simulink library "SDTlibV1"  (R2025b)
settings: Solver=VariableStepAuto  StartTime=0.0  StopTime=10.0  RelTol=1e-3
PreLoadFcn:
  | addpath(genpath('SDTfct'));
values from neighbouring files (symbols this model uses):
  pass = ra2DCMi(blk.ra)    [view_SDTlib_model.m]
undefined symbols (not defined in the file or in its folder): CMG, DAP0, DPa0, FSM, Ignew, InvDyn, InvDynAug, Jr, KIN, kinematic_model, LS, Mdyn, mnew, mp, OGnew, PMA, ra_norm, RWS, sig4, uls, ureal, uss, uw, XI
libraries: RCTblocks x470, $bdroot x4
(part 3 of 10)

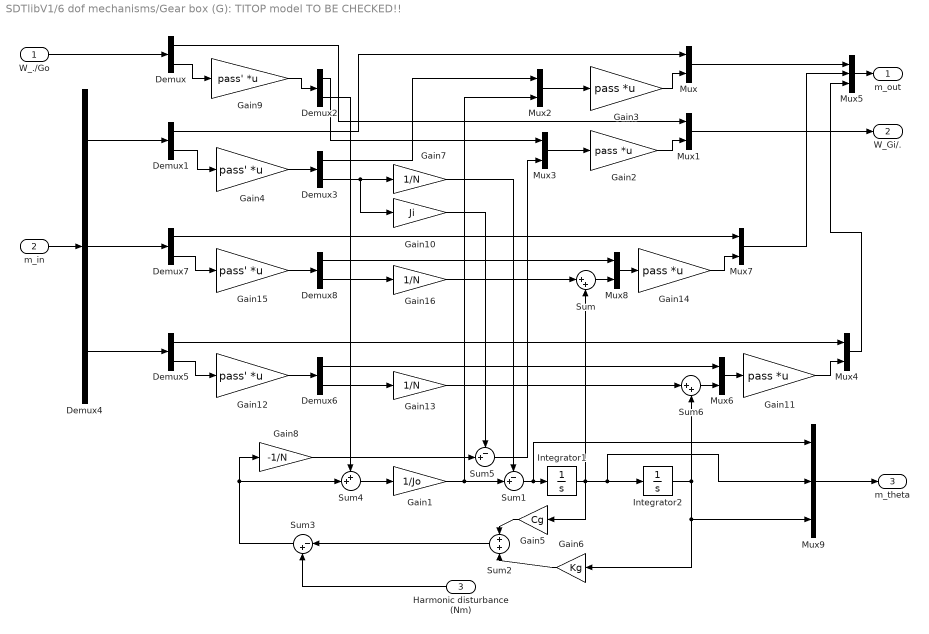
== system SDTlibV1/6 dof mechanisms/Gear box (G): TITOP model TO BE CHECKED!! ==
  W_./Go : Inport  PortDimensions=6
  m_in : Inport  Port=2  PortDimensions=18
  Harmonic disturbance (Nm) : Inport  Port=3
  Demux{,1,5,7} (4 alike) : Demux  Outputs=[3 3]
  Demux{2..3,6,8} (4 alike) : Demux  Outputs=[2 1]
  Demux4 : Demux  Outputs=[6 6 6]
  Gain1 : Gain  Gain=1/Jo
  Gain10 : Gain  Gain=Ji
  Gain{2..3,11,14} (4 alike) : Gain  Gain=pass  Multiplication=Matrix(K*u) (u vector)
  Gain{4,9,12,15} (4 alike) : Gain  Gain=pass'  Multiplication=Matrix(K*u) (u vector)
  Gain13 : Gain  Gain=1/N
  Gain16 : Gain  Gain=1/N
  Gain5 : Gain  Gain=Cg
  Gain6 : Gain  Gain=Kg
  Gain7 : Gain  Gain=1/N
  Gain8 : Gain  Gain=-1/N
  Integrator1 : Integrator
  Integrator2 : Integrator
  Mux{,1,4,7} (4 alike) : Mux  Inputs=[3 3]
  Mux{2..3,6,8} (4 alike) : Mux  Inputs=[2 1]
  Mux5 : Mux  Inputs=[6 6 6]
  Mux9 : Mux  Inputs=3
  Sum : Sum  Inputs=|++
  Sum1 : Sum  Inputs=-+|
  Sum2 : Sum
  Sum3 : Sum  Inputs=|-+
  Sum4 : Sum  Inputs=++|
  Sum5 : Sum  Inputs=-+|
  Sum6 : Sum  Inputs=|++
  m_out : Outport
  W_Gi/. : Outport  Port=2
  m_theta : Outport  Port=3
  wires:
  Mux1/1 -> W_Gi/./1
  Demux1/1 -> Mux/1
  Sum3/1 -> Sum4/2, Gain8/1
  Demux/1 -> Mux1/1
  Gain2/1 -> Mux1/2
  Integrator2/1 -> Mux9/3, Gain6/1, Sum6/2
  Demux/2 -> Gain9/1
  Gain1/1 -> Mux2/2, Sum1/2
  Sum2/1 -> Sum3/1
  Sum4/1 -> Gain1/1
  Gain5/1 -> Sum2/1
  Harmonic disturbance (Nm)/1 -> Sum3/2
  Gain6/1 -> Sum2/2
  Gain3/1 -> Mux/2
  Demux3/2 -> Gain10/1, Gain7/1
  Gain9/1 -> Demux2/1
  Demux2/2 -> Sum4/1
  Mux2/1 -> Gain3/1
  Demux1/2 -> Gain4/1
  Gain4/1 -> Demux3/1
  Mux3/1 -> Gain2/1
  Demux2/1 -> Mux3/1
  Demux3/1 -> Mux2/1
  W_./Go/1 -> Demux/1
  Gain7/1 -> Sum1/1
  Gain8/1 -> Sum5/2
  Sum5/1 -> Mux3/2
  Gain10/1 -> Sum5/1
  Demux4/1 -> Demux1/1
  m_in/1 -> Demux4/1
  Mux/1 -> Mux5/1
  Mux5/1 -> m_out/1
  Integrator1/1 -> Mux9/2, Integrator2/1, Gain5/1, Sum/2
  Demux8/1 -> Mux8/1
  Gain15/1 -> Demux8/1
  Gain14/1 -> Mux7/2
  Demux8/2 -> Gain16/1
  Demux4/2 -> Demux7/1
  Demux7/1 -> Mux7/1
  Demux7/2 -> Gain15/1
  Mux8/1 -> Gain14/1
  Gain16/1 -> Sum/1
  Mux7/1 -> Mux5/2
  Sum/1 -> Mux8/2
  Demux5/2 -> Gain12/1
  Demux6/1 -> Mux6/1
  Mux6/1 -> Gain11/1
  Demux5/1 -> Mux4/1
  Gain11/1 -> Mux4/2
  Gain13/1 -> Sum6/1
  Sum6/1 -> Mux6/2
  Gain12/1 -> Demux6/1
  Demux6/2 -> Gain13/1
  Demux4/3 -> Demux5/1
  Mux4/1 -> Mux5/3
  Mux9/1 -> m_theta/1
  Sum1/1 -> Mux9/1, Integrator1/1

== system SDTlibV1/6 dof mechanisms/Local Spring-Damper system  ==
  m_C : Inport  PortDimensions=18
  m_P : Inport  Port=2  PortDimensions=18
  Damping Matrix : RCTblocks/Uncertain State Space  Tag=USS  USystem=ss(D_O)  UValue=[]  X0=[]  uX0=[]
  Damping Matrix1 : RCTblocks/Uncertain State Space  Tag=USS  USystem=ss(K_O)  UValue=[]  X0=[]  uX0=[]
  Demux : Demux  Outputs=[6 6 6]
  Demux1 : Demux  Outputs=[6 6 6]
  Kinematic model between O and C : RCTblocks/Uncertain State Space  Tag=USS  USystem=ss(TAU_OC)  UValue=[]  X0=[]  uX0=[]
  Kinematic model between O and C' : RCTblocks/Uncertain State Space  Tag=USS  USystem=ss(TAU_OC')  UValue=[]  X0=[]  uX0=[]
  Kinematic model between O and C1 : RCTblocks/Uncertain State Space  Tag=USS  USystem=ss(TAU_OC)  UValue=[]  X0=[]  uX0=[]
  Kinematic model between O and P : RCTblocks/Uncertain State Space  Tag=USS  USystem=ss(TAU_OP)  UValue=[]  X0=[]  uX0=[]
  Kinematic model between O and P' : RCTblocks/Uncertain State Space  Tag=USS  USystem=ss(TAU_OP')  UValue=[]  X0=[]  uX0=[]
  Kinematic model between O and P1 : RCTblocks/Uncertain State Space  Tag=USS  USystem=ss(TAU_OP)  UValue=[]  X0=[]  uX0=[]
  Sum : Sum  Inputs=|+-
  Sum1 : Sum  Inputs=++|
  Sum2 : Sum  Inputs=|+-
  Terminator : Terminator
  Terminator1 : Terminator
  W(./s,C) : Outport  VectorParamsAs1DForOutWhenUnconnected=off
  W(s/.,P) : Outport  Port=2  VectorParamsAs1DForOutWhenUnconnected=off
  wires:
  Kinematic model between O and C'/1 -> W(./s,C)/1
  Kinematic model between O and P'/1 -> W(s/.,P)/1
  Sum/1 -> Damping Matrix/1
  Kinematic model between O and C/1 -> Sum/1
  Kinematic model between O and P/1 -> Sum/2
  Damping Matrix/1 -> Sum1/2
  Damping Matrix1/1 -> Sum1/1
  Sum2/1 -> Damping Matrix1/1
  Sum1/1 -> Kinematic model between O and C'/1, Kinematic model between O and P'/1
  m_P/1 -> Demux/1
  Demux/2 -> Kinematic model between O and P/1
  Demux/1 -> Terminator/1
  m_C/1 -> Demux1/1
  Demux1/1 -> Terminator1/1
  Demux1/2 -> Kinematic model between O and C/1
  Demux1/3 -> Kinematic model between O and C1/1
  Demux/3 -> Kinematic model between O and P1/1
  Kinematic model between O and C1/1 -> Sum2/1
  Kinematic model between O and P1/1 -> Sum2/2

== system SDTlibV1/6 dof mechanisms/PMA ==
  m_P : Inport
  u_PMA : Inport  Port=2
  Demux : Demux  Outputs=[6 12]
  Multi port rigid body : Subsystem  mask(Multi-port rigid body (6nx6n)){m=Mc-mp, Ig=IatG, OG=PG, n=2, numinv=1, OP1=[0;0;0], OP2=PG, OP3=[ureal('P3_y',1,'percent',10);0;0], OP4=[0;0;0], OP5=[0;0;0]}
      mask prompts: m "Mass (Kg)"; Ig "Inertia (at G, Kg m^2)"; OG "OG (3x1 vector, m)"; n "Number of ports"; numinv "Port to be inverted"; OP1 "OP1 (3x1 vector, m)"; OP2 "OP2 (3x1 vector, m)"; OP3 "OP3 (3x1 vector, m)"; OP4 "OP4 (3x1 vector, m)"; OP5 "OP5 (3x1 vector,m)"
      mask help:
      | 6nx6n dynamic model of a rigid body at n given points (ports) between wrenches applied at the n points (input) and acceleration twists at these points (output).
      |
      | 0: the reference point
      | G: the center of mass
      | Pi (i=1:n): the n given connection points (n<6).
      |
      | All parameters are expressed in the body frame.
      | Each parameter can be an uncertain parameter declared with "ureal"
      |
      | The 6x6 channel associated to one port can be inverted: then the input of this channel is the acceleration twist imposed at this point and the output is the wrench applied by this body.
      mask init:
      | MultiPortRigidBodyAug
      mask Help: web('Docmultiportrigidbody.html','-browser','-browser')
      mask TypeOptions n: 1 | 2 | 3 | 4 | 5
      mask TypeOptions numinv: 1 | 2 | 3 | 4 | 5
      mask DialogControl ParameterGroupVar Prompt: Main parameters
      mask DialogControl port1 Prompt: Port #1
      mask DialogControl port2 Prompt: #2
      mask DialogControl port3 Prompt: #3
      mask DialogControl port4 Prompt: #4
      mask DialogControl port5 Prompt: #5
      mask Display:
      | disp('Multi-port\n rigid body\n [18(n-1)+6]x[6(n-1)+18])')
      | if n==1,
      |     if numinv==1,
      |         port_label('input', 1,'m_P')
      |         port_label('output',1,'W_body/.,P')
      |     else
      |         port_label('input', 1,'W_./body,P')
      |         port_label('output',1,'m_P')
      |     end
      | else
      |     for ii=1:n
      |         if numinv==ii,
      |             port_label('output',ii,['W_body/.,P',num2str(ii)])
      |             port_label('input', ii,['m_P',num2str(ii)])
      |         else
      |             port_label('input', ii,['W_./body,P',num2str(ii)])
      |             port_label('output',ii,['m_P',num2str(ii)])
      |         end
      |     end
      | end
  Terminator : Terminator
  proof mass : Subsystem  mask(Mass-spring-model model(6x6)){v=v, m=mp, k=k, d=d}
      mask prompts: v "v (3x1 vector)"; m "mass (Kg)"; k "stiffness (N/m)"; d "damper (Ns/m)"
      mask help:
      | Simplified dynamic model of a spring-mass-damper model located at point P (connection point with the hub):
      | 6x6 transfer between acceleretion twist at P and wrench applied by the spring-mass system at P. The model is expressed in the (inherit) body frame.
      |
      | v: the direction vector of the spring-mass system.
      | Each parameter (except v) can be an uncertain parameter declared with "ureal"
      mask init:
      | pass=ra2DCMi(v);
      mask DialogControl ParameterGroupVar Prompt: Main parameters
      mask Display:
      | disp('1D \n mass-spring-damper \n model(6x6)')
      | port_label('input', 1, 'Xddot')
      | port_label('output', 1, 'W_body/.')
      | port_label('input', 2, 'u_PMA')
      | port_label('output', 2, 'x_PMA')
  W_body/.,P : Outport
  x_PMA : Outport  Port=2
  wires:
  Multi port rigid body/1(out1) -> W_body/.,P/1
  u_PMA/1 -> proof mass/2(u_PMA)
  m_P/1 -> Multi port rigid body/1(in1)
  proof mass/1(W_body/.) -> Multi port rigid body/2(in2)
  proof mass/2(x_PMA) -> x_PMA/1
  Multi port rigid body/2(out2) -> Demux/1
  Demux/1 -> proof mass/1(Xddot)
  Demux/2 -> Terminator/1

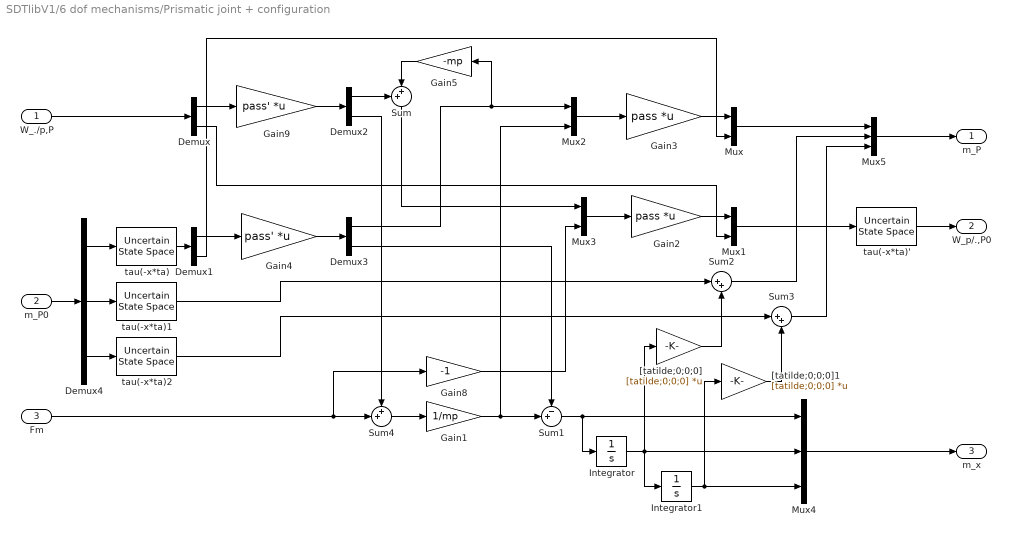
== system SDTlibV1/6 dof mechanisms/Prismatic joint + configuration ==
  W_./p,P : Inport  PortDimensions=6
  m_P0 : Inport  Port=2  PortDimensions=18
  Fm : Inport  Port=3  PortDimensions=1
  Demux : Demux  Outputs=[3 3]
  Demux1 : Demux  Outputs=[3 3]
  Demux2 : Demux  Outputs=[2 1]
  Demux3 : Demux  Outputs=[2 1]
  Demux4 : Demux  Outputs=[6 6 6]
  Gain1 : Gain  Gain=1/mp
  Gain2 : Gain  Gain=pass  Multiplication=Matrix(K*u) (u vector)
  Gain3 : Gain  Gain=pass  Multiplication=Matrix(K*u) (u vector)
  Gain4 : Gain  Gain=pass'  Multiplication=Matrix(K*u) (u vector)
  Gain5 : Gain  Gain=-mp
  Gain8 : Gain  Gain=-1
  Gain9 : Gain  Gain=pass'  Multiplication=Matrix(K*u) (u vector)
  Integrator : Integrator
  Integrator1 : Integrator
  Mux : Mux  Inputs=[3 3]
  Mux1 : Mux  Inputs=[3 3]
  Mux2 : Mux  Inputs=[2 1]
  Mux3 : Mux  Inputs=[2 1]
  Mux4 : Mux  Inputs=3
  Mux5 : Mux  Inputs=[6 6 6]
  Sum : Sum  Inputs=++|
  Sum1 : Sum  Inputs=-+|
  Sum2 : Sum  Inputs=|++
  Sum3 : Sum  Inputs=|++
  Sum4 : Sum  Inputs=++|
  "[tatilde;0;0;0]" : Gain  Gain=[tatilde;0;0;0]  Multiplication=Matrix(K*u) (u vector)
  "[tatilde;0;0;0]1" : Gain  Gain=[tatilde;0;0;0]  Multiplication=Matrix(K*u) (u vector)
  tau(-x*ta) : RCTblocks/Uncertain State Space  Tag=USS  USystem=tau_x  UValue=[]  X0=[]  uX0=[]
  tau(-x*ta)' : RCTblocks/Uncertain State Space  Tag=USS  USystem=tau_x'  UValue=[]  X0=[]  uX0=[]
  tau(-x*ta)1 : RCTblocks/Uncertain State Space  Tag=USS  USystem=tau_x  UValue=[]  X0=[]  uX0=[]
  tau(-x*ta)2 : RCTblocks/Uncertain State Space  Tag=USS  USystem=tau_x  UValue=[]  X0=[]  uX0=[]
  m_P : Outport  VectorParamsAs1DForOutWhenUnconnected=off
  W_p/.,P0 : Outport  Port=2  VectorParamsAs1DForOutWhenUnconnected=off
  m_x : Outport  Port=3  VectorParamsAs1DForOutWhenUnconnected=off
  wires:
  Mux1/1 -> tau(-x*ta)'/1
  Fm/1 -> Gain8/1, Sum4/2
  Gain1/1 -> Mux2/2, Sum1/2
  Sum4/1 -> Gain1/1
  Demux3/2 -> Sum1/1
  Gain9/1 -> Demux2/1
  Mux2/1 -> Gain3/1
  Gain4/1 -> Demux3/1
  Mux3/1 -> Gain2/1
  Gain8/1 -> Mux3/2
  Demux3/1 -> Gain5/1, Mux2/1
  W_./p,P/1 -> Demux/1
  Demux/1 -> Gain9/1
  Demux2/2 -> Sum4/1
  Gain2/1 -> Mux1/1
  Demux/2 -> Mux1/2
  Demux1/1 -> Gain4/1
  Demux1/2 -> Mux/2
  Gain3/1 -> Mux/1
  tau(-x*ta)/1 -> Demux1/1
  tau(-x*ta)'/1 -> W_p/.,P0/1
  Demux2/1 -> Sum/1
  Gain5/1 -> Sum/2
  Sum/1 -> Mux3/1
  Demux4/1 -> tau(-x*ta)/1
  Demux4/2 -> tau(-x*ta)1/1
  Demux4/3 -> tau(-x*ta)2/1
  m_P0/1 -> Demux4/1
  Mux4/1 -> m_x/1
  "[tatilde;0;0;0]1"/1 -> Sum3/2
  "[tatilde;0;0;0]"/1 -> Sum2/2
  Integrator1/1 -> "[tatilde;0;0;0]1"/1, Mux4/3
  Integrator/1 -> "[tatilde;0;0;0]"/1, Mux4/2, Integrator1/1
  Sum1/1 -> Integrator/1, Mux4/1
  tau(-x*ta)1/1 -> Sum2/1
  tau(-x*ta)2/1 -> Sum3/1
  Mux/1 -> Mux5/1
  Sum2/1 -> Mux5/2
  Sum3/1 -> Mux5/3
  Mux5/1 -> m_P/1

== system SDTlibV1/6 dof mechanisms/RW ==
  m : Inport  PortDimensions=18
  u (Nm) : Inport  Port=2  PortDimensions=1
  Demux : Demux  Outputs=[3 3]
  Demux1 : Demux  Outputs=[2 1]
  Demux2 : Demux  Outputs=[6 6 6]
  Demux3 : Demux  Outputs=[3 3]
  Demux4 : Demux  Outputs=[2 1]
  Gain : Gain  Gain=-1
  Gain1 : Gain  Gain=pass'  Multiplication=Matrix(K*u) (u vector)
  Gain10 : Gain  Gain=pass'  Multiplication=Matrix(K*u) (u vector)
  Gain2 : Gain  Gain=pass  Multiplication=Matrix(K*u) (u vector)
  Gain3 : Gain  Gain=m*eye(3)  Multiplication=Matrix(K*u) (u vector)
  Gain4 : Gain  Gain=diag([Ir Ir 0])  Multiplication=Matrix(K*u) (u vector)
  Gain5 : Gain  Gain=Tau_GP  Multiplication=Matrix(K*u) (u vector)
  Gain6 : Gain  Gain=[0 Iw;-Iw 0]  Multiplication=Matrix(K*u) (u vector)
  Gain7 : Gain  Gain=1/Iw
  Gain8 : Gain  Gain=-Tau_GP'  Multiplication=Matrix(K*u) (u vector)
  Gain9 : Gain  Gain=Tau_GP  Multiplication=Matrix(K*u) (u vector)
  Mux : Mux  Inputs=[3 3]
  Mux2 : Mux  Inputs=[2 1]
  Omega : RCTblocks/Uncertain State Space  Tag=USS  USystem=uss(Omega*eye(2))  UValue=[]  X0=[]  uX0=[]
  Sum : Sum
  Sum1 : Sum  Inputs=-+|
  Terminator{,1..3} (4 alike) : Terminator
  W_body/. : Outport  VectorParamsAs1DForOutWhenUnconnected=off
  Omega dot (rad/s^2) : Outport  Port=2  PortDimensions=1  VectorParamsAs1DForOutWhenUnconnected=off
  wires:
  Gain3/1 -> Mux/1
  Gain2/1 -> Mux/2
  Demux/1 -> Gain3/1
  Demux/2 -> Gain1/1
  Gain4/1 -> Sum/1
  Sum/1 -> Gain2/1
  Gain1/1 -> Demux1/1, Gain4/1
  Demux4/1 -> Gain6/1
  Gain6/1 -> Omega/1
  Gain8/1 -> W_body/./1
  Mux/1 -> Gain8/1
  Gain9/1 -> Demux/1
  u (Nm)/1 -> Gain/1
  Sum1/1 -> Omega dot (rad/s^2)/1
  Gain7/1 -> Sum1/2
  Gain/1 -> Mux2/2, Gain7/1
  Omega/1 -> Mux2/1
  Mux2/1 -> Sum/2
  Demux2/1 -> Gain9/1
  m/1 -> Demux2/1
  Demux2/2 -> Gain5/1
  Gain5/1 -> Demux3/1
  Demux3/2 -> Gain10/1
  Demux3/1 -> Terminator/1
  Demux2/3 -> Terminator1/1
  Demux1/2 -> Sum1/1
  Demux1/1 -> Terminator2/1
  Gain10/1 -> Demux4/1
  Demux4/2 -> Terminator3/1

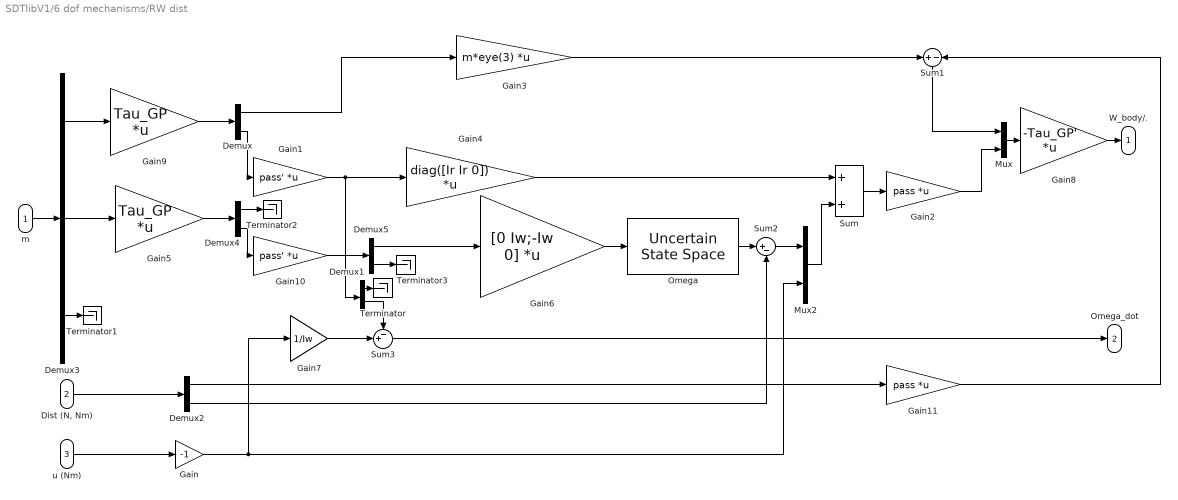
== system SDTlibV1/6 dof mechanisms/RW dist ==
  m : Inport  PortDimensions=18
  "Dist (N, Nm)    " : Inport  Port=2
  u (Nm) : Inport  Port=3  PortDimensions=1
  Demux : Demux  Outputs=[3 3]
  Demux1 : Demux  Outputs=[2 1]
  Demux2 : Demux  Outputs=[3 2]
  Demux3 : Demux  Outputs=[6 6 6]
  Demux4 : Demux  Outputs=[3 3]
  Demux5 : Demux  Outputs=[2 1]
  Gain : Gain  Gain=-1
  Gain1 : Gain  Gain=pass'  Multiplication=Matrix(K*u) (u vector)
  Gain10 : Gain  Gain=pass'  Multiplication=Matrix(K*u) (u vector)
  Gain11 : Gain  Gain=pass  Multiplication=Matrix(K*u) (u vector)
  Gain2 : Gain  Gain=pass  Multiplication=Matrix(K*u) (u vector)
  Gain3 : Gain  Gain=m*eye(3)  Multiplication=Matrix(K*u) (u vector)
  Gain4 : Gain  Gain=diag([Ir Ir 0])  Multiplication=Matrix(K*u) (u vector)
  Gain5 : Gain  Gain=Tau_GP  Multiplication=Matrix(K*u) (u vector)
  Gain6 : Gain  Gain=[0 Iw;-Iw 0]  Multiplication=Matrix(K*u) (u vector)
  Gain7 : Gain  Gain=1/Iw
  Gain8 : Gain  Gain=-Tau_GP'  Multiplication=Matrix(K*u) (u vector)
  Gain9 : Gain  Gain=Tau_GP  Multiplication=Matrix(K*u) (u vector)
  Mux : Mux  Inputs=[3 3]
  Mux2 : Mux  Inputs=[2 1]
  Omega : RCTblocks/Uncertain State Space  Tag=USS  USystem=uss(Omega*eye(2))  UValue=[]  X0=[]  uX0=[]
  Sum : Sum
  Sum1 : Sum  Inputs=+-
  Sum2 : Sum  Inputs=|+-
  Sum3 : Sum  Inputs=-+|
  Terminator{,1..3} (4 alike) : Terminator
  W_body/. : Outport  VectorParamsAs1DForOutWhenUnconnected=off
  Omega_dot : Outport  Port=2  PortDimensions=1  VectorParamsAs1DForOutWhenUnconnected=off
  wires:
  Sum3/1 -> Omega_dot/1
  Gain7/1 -> Sum3/2
  Mux2/1 -> Sum/2
  Sum2/1 -> Mux2/1
  Omega/1 -> Sum2/1
  Gain/1 -> Gain7/1, Mux2/2
  u (Nm)/1 -> Gain/1
  Sum1/1 -> Mux/1
  Gain11/1 -> Sum1/2
  Gain3/1 -> Sum1/1
  Demux2/2 -> Sum2/2
  "Dist (N, Nm)    "/1 -> Demux2/1
  Demux2/1 -> Gain11/1
  Gain9/1 -> Demux/1
  Mux/1 -> Gain8/1
  Gain8/1 -> W_body/./1
  Gain6/1 -> Omega/1
  Demux5/1 -> Gain6/1
  Gain1/1 -> Gain4/1, Demux1/1
  Sum/1 -> Gain2/1
  Gain4/1 -> Sum/1
  Demux/2 -> Gain1/1
  Demux/1 -> Gain3/1
  Gain2/1 -> Mux/2
  Demux3/1 -> Gain9/1
  m/1 -> Demux3/1
  Demux3/2 -> Gain5/1
  Demux1/2 -> Sum3/1
  Demux1/1 -> Terminator/1
  Demux3/3 -> Terminator1/1
  Demux4/2 -> Gain10/1
  Gain5/1 -> Demux4/1
  Demux4/1 -> Terminator2/1
  Gain10/1 -> Demux5/1
  Demux5/2 -> Terminator3/1

== system SDTlibV1/6 dof mechanisms/RW_NL ==
  m : Inport  PortDimensions=18
  u (Nm) : Inport  Port=2  PortDimensions=1
  Demux : Demux  Outputs=[3 3]
  Demux1 : Demux  Outputs=[2 1]
  Demux2 : Demux  Outputs=[6 6 6]
  Demux3 : Demux  Outputs=[3 3]
  Demux4 : Demux  Outputs=[2 1]
  Gain : Gain  Gain=-1
  Gain1 : Gain  Gain=pass'  Multiplication=Matrix(K*u) (u vector)
  Gain10 : Gain  Gain=Tau_GP  Multiplication=Matrix(K*u) (u vector)
  Gain2 : Gain  Gain=pass  Multiplication=Matrix(K*u) (u vector)
  Gain3 : Gain  Gain=m*eye(3)  Multiplication=Matrix(K*u) (u vector)
  Gain4 : Gain  Gain=diag([Ir Ir 0])  Multiplication=Matrix(K*u) (u vector)
  Gain5 : Gain  Gain=pass'  Multiplication=Matrix(K*u) (u vector)
  Gain6 : Gain  Gain=[0 Iw;-Iw 0]  Multiplication=Matrix(K*u) (u vector)
  Gain7 : Gain  Gain=1/Iw
  Gain8 : Gain  Gain=-Tau_GP'  Multiplication=Matrix(K*u) (u vector)
  Gain9 : Gain  Gain=Tau_GP  Multiplication=Matrix(K*u) (u vector)
  Integrator2 : Integrator  InitialCondition=Omega
  Mux : Mux  Inputs=[3 3]
  Mux2 : Mux  Inputs=[2 1]
  Product : Product
  Sum : Sum
  Sum1 : Sum  Inputs=-+
  Terminator{,1..3} (4 alike) : Terminator
  W_body/. : Outport  VectorParamsAs1DForOutWhenUnconnected=off
  Omega : Outport  Port=2  PortDimensions=1  VectorParamsAs1DForOutWhenUnconnected=off
  wires:
  Mux2/1 -> Sum/2
  Product/1 -> Mux2/1
  Demux1/2 -> Sum1/1
  Gain7/1 -> Sum1/2
  Sum1/1 -> Integrator2/1
  Gain/1 -> Gain7/1, Mux2/2
  Integrator2/1 -> Product/2, Omega/1
  u (Nm)/1 -> Gain/1
  Gain9/1 -> Demux/1
  Mux/1 -> Gain8/1
  Gain8/1 -> W_body/./1
  Gain6/1 -> Product/1
  Demux4/1 -> Gain6/1
  Gain1/1 -> Gain4/1, Demux1/1
  Sum/1 -> Gain2/1
  Gain4/1 -> Sum/1
  Demux/2 -> Gain1/1
  Demux/1 -> Gain3/1
  Gain2/1 -> Mux/2
  Gain3/1 -> Mux/1
  Demux2/1 -> Gain9/1
  m/1 -> Demux2/1
  Demux1/1 -> Terminator/1
  Demux2/3 -> Terminator1/1
  Gain5/1 -> Demux4/1
  Gain10/1 -> Demux3/1
  Demux3/2 -> Gain5/1
  Demux2/2 -> Gain10/1
  Demux3/1 -> Terminator2/1
  Demux4/2 -> Terminator3/1

== system SDTlibV1/6 dof mechanisms/Revolute joint ==
  W_./r_out : Inport  PortDimensions=6
  m_in : Inport  Port=2  PortDimensions=18
  Cm : Inport  Port=3  PortDimensions=1
  Demux : Demux  Outputs=[3 3]
  Demux1 : Demux  Outputs=[3 3]
  Demux2 : Demux  Outputs=[2 1]
  Demux3 : Demux  Outputs=[2 1]
  Demux4 : Demux  Outputs=[6 6 6]
  Gain1 : Gain  Gain=1/Jr
  Gain2 : Gain  Gain=pass  Multiplication=Matrix(K*u) (u vector)
  Gain3 : Gain  Gain=pass  Multiplication=Matrix(K*u) (u vector)
  Gain4 : Gain  Gain=pass'  Multiplication=Matrix(K*u) (u vector)
  Gain8 : Gain  Gain=-1
  Gain9 : Gain  Gain=pass'  Multiplication=Matrix(K*u) (u vector)
  Integrator : Integrator
  Integrator1 : Integrator
  Mux : Mux  Inputs=[3 3]
  Mux1 : Mux  Inputs=[3 3]
  Mux2 : Mux  Inputs=[2 1]
  Mux3 : Mux  Inputs=[2 1]
  Mux4 : Mux  Inputs=3
  Mux5 : Mux  Inputs=[6 6 6]
  Sum : Sum  Inputs=|++
  Sum1 : Sum  Inputs=-+|
  Sum2 : Sum  Inputs=|++
  Sum4 : Sum  Inputs=++|
  "[0;0;0;ran]" : Gain  Gain=[zeros(3,1);ran]  Multiplication=Matrix(K*u) (u vector)
  "[0;0;0;ran]1" : Gain  Gain=[zeros(3,1);ran]  Multiplication=Matrix(K*u) (u vector)
  m_out : Outport  VectorParamsAs1DForOutWhenUnconnected=off
  W_r_in/. : Outport  Port=2  VectorParamsAs1DForOutWhenUnconnected=off
  m_theta : Outport  Port=3  VectorParamsAs1DForOutWhenUnconnected=off
  wires:
  Mux1/1 -> W_r_in/./1
  Demux1/1 -> Mux/1
  Cm/1 -> Gain8/1, Sum4/2
  Demux/1 -> Mux1/1
  Gain2/1 -> Mux1/2
  Sum1/1 -> Integrator/1, Mux4/1
  Demux/2 -> Gain9/1
  Gain1/1 -> Mux2/2, Sum1/2
  Sum4/1 -> Gain1/1
  Gain3/1 -> Mux/2
  Demux3/2 -> Sum1/1
  Gain9/1 -> Demux2/1
  Demux2/2 -> Sum4/1
  Mux2/1 -> Gain3/1
  Demux1/2 -> Gain4/1
  Gain4/1 -> Demux3/1
  Mux3/1 -> Gain2/1
  Gain8/1 -> Mux3/2
  Demux2/1 -> Mux3/1
  Demux3/1 -> Mux2/1
  W_./r_out/1 -> Demux/1
  Demux4/1 -> Demux1/1
  m_in/1 -> Demux4/1
  Integrator/1 -> "[0;0;0;ran]"/1, Mux4/2, Integrator1/1
  Integrator1/1 -> "[0;0;0;ran]1"/1, Mux4/3
  Mux4/1 -> m_theta/1
  Demux4/2 -> Sum/1
  "[0;0;0;ran]"/1 -> Sum/2
  "[0;0;0;ran]1"/1 -> Sum2/2
  Demux4/3 -> Sum2/1
  Mux/1 -> Mux5/1
  Sum/1 -> Mux5/2
  Sum2/1 -> Mux5/3
  Mux5/1 -> m_out/1

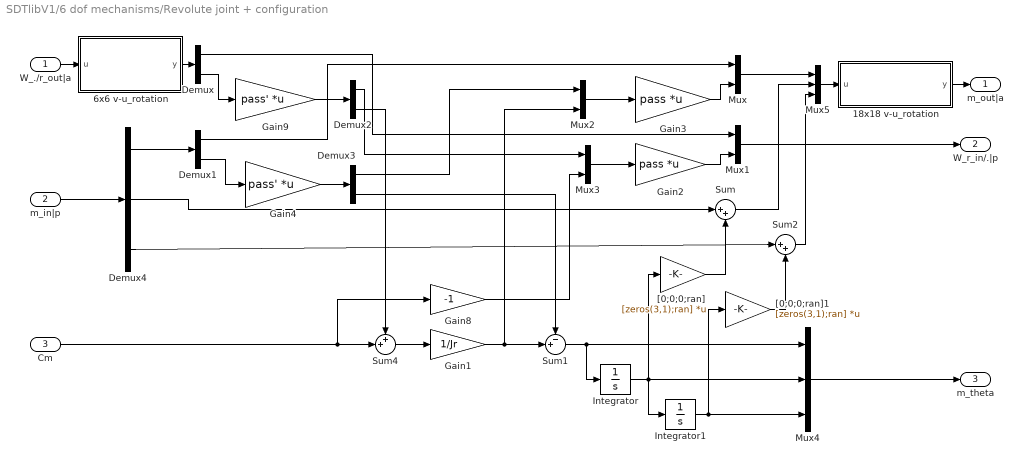
== system SDTlibV1/6 dof mechanisms/Revolute joint + configuration ==
  W_./r_out|a : Inport  PortDimensions=6
  m_in|p : Inport  Port=2  PortDimensions=18
  Cm : Inport  Port=3  PortDimensions=1
  18x18 v-u_rotation : Subsystem  mask(18x18 rotation matrix (around a given axis)){ra=ra, theta=theta, transp=on}
      mask prompts: ra "Rotation axis (3x1 vector)"; theta "Angle (rad)"; transp "Matrix transposed"
      mask help:
      | For 6 d.o.f. body motion vector (3 translations and 3 rotations, acceleration velocities and positions), this block Implement the 18x18 rotation matrix (or its transposed)  for a given angle around a given axis.
      |
      | Angle  (rad) can be an uncertain parameter declared with "ureal" with mode 'Range'
      | Ex: ureal('NAME',0,'Range',[-pi pi])
      | Then, ULINEARIZE will provide a model involving the block named "tan_NAME_div4".
      mask init:
      | vUrotation3x3
      mask Help: web('Doc6vurotation.html','-browser','-browser')
      mask Display:
      | disp('v-rot\n18x18')
      | if transp
      |     port_label('input', 1, '[.]_R1')
      |     port_label('output', 1, '[.]_R2')
      | else
      |     port_label('input', 1, '[.]_R2')
      |     port_label('output', 1, '[.]_R1')
      | end
  6x6 v-u_rotation : Subsystem  mask(6x6 rotation matrix (around a given axis)){ra=ra, theta=theta, transp=off}
      mask prompts: ra "Rotation axis (3x1 vector)"; theta "Angle (rad)"; transp "Matrix transposed"
      mask help:
      | For 6 d.o.f. body motion (3 translations and 3 rotations), this block Implement the 6x6 rotation matrix (or its transposed) for a given angle around a given axis.
      |
      | Angle  (rad) can be an uncertain parameter declared with "ureal" with mode 'Range'
      | Ex: ureal('NAME',0,'Range',[-pi pi])
      | Then, ULINEARIZE will provide a model involving the block named "tan_NAME_div4".
      mask init:
      | vUrotation3x3
      mask Help: web('Doc6vurotation.html','-browser','-browser')
      mask Display:
      | disp('v-rot\n6x6')
      | if transp
      |     port_label('input', 1, '[.]_R1')
      |     port_label('output', 1, '[.]_R2')
      | else
      |     port_label('input', 1, '[.]_R2')
      |     port_label('output', 1, '[.]_R1')
      | end
  Demux : Demux  Outputs=[3 3]
  Demux1 : Demux  Outputs=[3 3]
  Demux2 : Demux  Outputs=[2 1]
  Demux3 : Demux  Outputs=[2 1]
  Demux4 : Demux  Outputs=[6 6 6]
  Gain1 : Gain  Gain=1/Jr
  Gain2 : Gain  Gain=pass  Multiplication=Matrix(K*u) (u vector)
  Gain3 : Gain  Gain=pass  Multiplication=Matrix(K*u) (u vector)
  Gain4 : Gain  Gain=pass'  Multiplication=Matrix(K*u) (u vector)
  Gain8 : Gain  Gain=-1
  Gain9 : Gain  Gain=pass'  Multiplication=Matrix(K*u) (u vector)
  Integrator : Integrator
  Integrator1 : Integrator
  Mux : Mux  Inputs=[3 3]
  Mux1 : Mux  Inputs=[3 3]
  Mux2 : Mux  Inputs=[2 1]
  Mux3 : Mux  Inputs=[2 1]
  Mux4 : Mux  Inputs=3
  Mux5 : Mux  Inputs=[6 6 6]
  Sum : Sum  Inputs=|++
  Sum1 : Sum  Inputs=-+|
  Sum2 : Sum  Inputs=|++
  Sum4 : Sum  Inputs=++|
  "[0;0;0;ran]" : Gain  Gain=[zeros(3,1);ran]  Multiplication=Matrix(K*u) (u vector)
  "[0;0;0;ran]1" : Gain  Gain=[zeros(3,1);ran]  Multiplication=Matrix(K*u) (u vector)
  m_out|a : Outport  VectorParamsAs1DForOutWhenUnconnected=off
  W_r_in/.|p : Outport  Port=2  VectorParamsAs1DForOutWhenUnconnected=off
  m_theta : Outport  Port=3  VectorParamsAs1DForOutWhenUnconnected=off
  wires:
  18x18 v-u_rotation/1(y) -> m_out|a/1
  6x6 v-u_rotation/1(y) -> Demux/1
  Demux3/1 -> Mux2/1
  Demux2/1 -> Mux3/1
  Gain8/1 -> Mux3/2
  Mux3/1 -> Gain2/1
  Gain4/1 -> Demux3/1
  Demux1/2 -> Gain4/1
  Mux2/1 -> Gain3/1
  Demux2/2 -> Sum4/1
  Gain9/1 -> Demux2/1
  Demux3/2 -> Sum1/1
  Gain3/1 -> Mux/2
  Sum4/1 -> Gain1/1
  Gain1/1 -> Sum1/2, Mux2/2
  Demux/2 -> Gain9/1
  Gain2/1 -> Mux1/2
  Demux/1 -> Mux1/1
  Cm/1 -> Sum4/2, Gain8/1
  Demux1/1 -> Mux/1
  Mux1/1 -> W_r_in/.|p/1
  W_./r_out|a/1 -> 6x6 v-u_rotation/1(u)
  Demux4/1 -> Demux1/1
  m_in|p/1 -> Demux4/1
  Integrator/1 -> "[0;0;0;ran]"/1, Mux4/2, Integrator1/1
  Mux4/1 -> m_theta/1
  Sum1/1 -> Integrator/1, Mux4/1
  Integrator1/1 -> "[0;0;0;ran]1"/1, Mux4/3
  "[0;0;0;ran]"/1 -> Sum/2
  "[0;0;0;ran]1"/1 -> Sum2/2
  Demux4/2 -> Sum/1
  Demux4/3 -> Sum2/1
  Mux/1 -> Mux5/1
  Mux5/1 -> 18x18 v-u_rotation/1(u)
  Sum/1 -> Mux5/2
  Sum2/1 -> Mux5/3

== system SDTlibV1/6 dof mechanisms/u_sloshing ==
  m : Inport  PortDimensions=18
  -m1 : RCTblocks/Uncertain State Space  Tag=USS  USystem=uss(-m*eye(3))  UValue=[]  X0=[]  uX0=[]
  2*xi : RCTblocks/Uncertain State Space  Tag=USS  USystem=uss(2*xi)  UValue=[]  X0=[]  uX0=[]
  Add1 : Sum
  Add3 : Sum  Inputs=+-
  Demux : Demux  Outputs=[3 3]
  Demux1 : Demux  Outputs=[2 1]
  Demux2 : Demux  Outputs=[6 12]
  Gain2 : Gain  Gain=pass'  Multiplication=Matrix(K*u) (u vector)
  Gain3 : Gain  Gain=pass  Multiplication=Matrix(K*u) (u vector)
  Ground : Ground
  Integrator : Integrator
  Integrator1 : Integrator
  Mux : Mux  Inputs=[2 1]
  Mux1 : Mux  Inputs=[3 3]
  Terminator : Terminator
  Terminator1 : Terminator
  omega : RCTblocks/Uncertain State Space  Tag=USS  USystem=uss(w)  UValue=[]  X0=[]  uX0=[]
  "omega_ " : RCTblocks/Uncertain State Space  Tag=USS  USystem=uss(w)  UValue=[]  X0=[]  uX0=[]
  Wbody/. : Outport  PortDimensions=6  VectorParamsAs1DForOutWhenUnconnected=off
  wires:
  Gain2/1 -> Demux1/1
  Demux/1 -> Gain2/1
  Demux/2 -> Terminator/1
  Ground/1 -> Mux1/2
  Gain3/1 -> Mux1/1
  Mux1/1 -> Wbody/./1
  2*xi/1 -> Add1/2
  Add1/1 -> omega/1
  Integrator1/1 -> "omega_ "/1  "-dx"
  Integrator/1 -> Integrator1/1, 2*xi/1  "-dx dot"
  "omega_ "/1 -> Add1/1
  Add3/1 -> Integrator/1  "-dx ddot"
  Demux1/2 -> Add3/1  "x_P ddot"
  -m1/1 -> Gain3/1
  Mux/1 -> -m1/1
  omega/1 -> Mux/2, Add3/2
  Demux1/1 -> Mux/1
  m/1 -> Demux2/1
  Demux2/2 -> Terminator1/1
  Demux2/1 -> Demux/1  "[ Xddot(P) ]/Rb"

== system SDTlibV1/Predefined subsystems/1 port flexible body + revolute joint ==
  m : Inport  PortDimensions=18
  Cm : Inport  Port=2  PortDimensions=1
  2*xi diagonal matrix : RCTblocks/Uncertain State Space  Tag=USS  USystem=uss(2*XI)  UValue=[]  X0=[]  uX0=[]
  Add : Sum  Inputs=--
  Add1 : Sum
  Add2 : Sum  Inputs=+-
  DAP0 : RCTblocks/Uncertain State Space  Tag=USS  USystem=uss(DAP0)  UValue=[]  X0=[]  uX0=[]
  Demux : Demux  Outputs=[6 12]
  Integrator : Integrator
  Integrator1 : Integrator
  Revolute joint + configuration : Subsystem  mask(Revolute joint){ra=ra, Jr=Jr, theta=theta}
      mask prompts: ra "Direction of the joint in the local frame (3x1 vector)"; Jr "Rotor inertia (kg.m^2)"; theta "Angular configuration (rad)"
      mask help:
      | This block implement the TITOP model of of a revolute joint.
      | The last channel is the transfer between the torque applied inside the joint by the input shaft to the output shaft and the relative angular acceleration of the output shaft w.r.t the input shaft.
      |
      | Angular configuration can be a vayring parameter: Ex:
      | ureal('NAME',0,'Range',[-pi pi])
      |
      | Then, ULINEARIZE will provide a model involving the block named "tan_NAME_div4";
      mask init:
      | pass=ra2DCMi(ra);
      | ran=[ra(1);ra(2);ra(3)]/norm(ra);
      mask Help: web('DocRevoluteJoint_configuration.html','-browser','-browser')
      mask Display:
      | disp('Revolute joint\nTITOP model\n+ angle configuration')
      | port_label('input', 1, 'W_./r_out|a')
      | port_label('output', 1, 'm_out|a')
      | port_label('input', 2, 'm_in|p')
      | port_label('output', 2, 'W_r_in/.|p')
      | port_label('input', 3, 'Cm')
      | port_label('output', 3, 'm_\theta','interpreter','tex')
  Terminator : Terminator
  "[Lp] ' Ra" : RCTblocks/Uncertain State Space  Tag=USS  USystem=uss(uls')  UValue=[]  X0=[]  uX0=[]
  "[Lp] Ra" : RCTblocks/Uncertain State Space  Tag=USS  USystem=uss(uls)  UValue=[]  X0=[]  uX0=[]
  omega diagonal matrix : RCTblocks/Uncertain State Space  Tag=USS  USystem=uss(diag(uw))  UValue=[]  X0=[]  uX0=[]
  omega diagonal matrix. : RCTblocks/Uncertain State Space  Tag=USS  USystem=uss(diag(uw))  UValue=[]  X0=[]  uX0=[]
  W_body/. : Outport  VectorParamsAs1DForOutWhenUnconnected=off
  theta_ddot : Outport  Port=2  VectorParamsAs1DForOutWhenUnconnected=off
  wires:
  Add2/1 -> Revolute joint + configuration/1(W_./r_out|a)  "[ F(A/P,p) ]/Ra"
  omega diagonal matrix/1 -> Add/1, "[Lp] ' Ra"/1
  "[Lp] Ra"/1 -> Add/2
  2*xi diagonal matrix/1 -> Add1/2
  Add1/1 -> omega diagonal matrix/1
  Add/1 -> Integrator/1  "eta dot dot"
  Integrator1/1 -> omega diagonal matrix./1  "eta"
  Integrator/1 -> Integrator1/1, 2*xi diagonal matrix/1  "eta dot"
  omega diagonal matrix./1 -> Add1/1
  "[Lp] ' Ra"/1 -> Add2/1
  DAP0/1 -> Add2/2
  m/1 -> Revolute joint + configuration/2(m_in|p)
  Revolute joint + configuration/2(W_r_in/.|p) -> W_body/./1
  Cm/1 -> Revolute joint + configuration/3(Cm)
  Revolute joint + configuration/3(m_theta) -> theta_ddot/1
  Revolute joint + configuration/1(m_out|a) -> Demux/1
  Demux/1 -> "[Lp] Ra"/1, DAP0/1  "[ Xddot(p) ]/Ra"
  Demux/2 -> Terminator/1

== system SDTlibV1/Predefined subsystems/Multi port rigid body + prismatic joint ==
  m_P1 : Inport
  Fm : Inport  Port=2
  W_./body,P2 : Inport  Port=3
  W_./body,P3 : Inport  Port=4
  Multi port rigid body : Subsystem  mask(Multi-port rigid body (6nx6n)){m=mnew, Ig=Ignew, OG=OGnew, n=3, numinv=1, OP1=[0;0;0], OP2=[0;0;0], OP3=[0;0;0], OP4=[0;0;1], OP5=[0;0;0]}
      mask prompts: m "Mass (Kg)"; Ig "Inertia (at G, Kg m^2)"; OG "OG (3x1 vector, m)"; n "Number of ports"; numinv "Port to be inverted"; OP1 "OP1 (3x1 vector, m)"; OP2 "OP2 (3x1 vector, m)"; OP3 "OP3 (3x1 vector, m)"; OP4 "OP4 (3x1 vector, m)"; OP5 "OP5 (3x1 vector,m)"
      mask help:
      | 6nx6n dynamic model of a rigid body at n given points (ports) between wrenches applied at the n points (input) and acceleration twists at these points (output).
      |
      | 0: the reference point
      | G: the center of mass
      | Pi (i=1:n): the n given connection points (n<6).
      |
      | All parameters are expressed in the body frame.
      | Each parameter can be an uncertain parameter declared with "ureal"
      |
      | The 6x6 channel associated to one port can be inverted: then the input of this channel is the acceleration twist imposed at this point and the output is the wrench applied by this body.
      mask init:
      | MultiPortRigidBodyAug
      mask Help: web('Docmultiportrigidbody.html','-browser','-browser')
      mask TypeOptions n: 1 | 2 | 3 | 4 | 5
      mask TypeOptions numinv: 1 | 2 | 3 | 4 | 5
      mask DialogControl ParameterGroupVar Prompt: Main parameters
      mask DialogControl port1 Prompt: Port #1
      mask DialogControl port2 Prompt: #2
      mask DialogControl port3 Prompt: #3
      mask DialogControl port4 Prompt: #4
      mask DialogControl port5 Prompt: #5
      mask Display:
      | disp('Multi-port\n rigid body\n [18(n-1)+6]x[6(n-1)+18])')
      | if n==1,
      |     if numinv==1,
      |         port_label('input', 1,'m_P')
      |         port_label('output',1,'W_body/.,P')
      |     else
      |         port_label('input', 1,'W_./body,P')
      |         port_label('output',1,'m_P')
      |     end
      | else
      |     for ii=1:n
      |         if numinv==ii,
      |             port_label('output',ii,['W_body/.,P',num2str(ii)])
      |             port_label('input', ii,['m_P',num2str(ii)])
      |         else
      |             port_label('input', ii,['W_./body,P',num2str(ii)])
      |             port_label('output',ii,['m_P',num2str(ii)])
      |         end
      |     end
      | end
  Prismatic joint + configuration : Subsystem  mask(Prismatic joint){ta=ta, mp=mp, x=x}
      mask prompts: ta "Direction of the joint in the local frame (3x1 vector)"; mp "Output slider mass (kg)"; x "Linear configuration (m)"
      mask help:
      | This block implement the TITOP model of a prismatic joint.
      | The last channel is the transfer between the force applied inside the joint by the input slider to the output slider and the relative linearr acceleration of the output slider w.r.t the input slider.
      |
      | Linear configuration can be a vayring parameter: Ex:
      | ureal('NAME',0,'Range',[-0.2 0.2])
      mask init:
      | pass=ra2DCMi(ta);
      | tatilde=[ta(1);ta(2);ta(3)]/norm(ta);
      | tau_x=kinematic_model(x*tatilde,[0;0;0]);
      mask Help: web('DocPrismatixJoint.html','-browser','-browser')
      mask Display:
      | disp('Prismatic joint\nTITOP model\n+ linear configuration')
      | port_label('input', 1, 'W_./p,P')
      | port_label('output', 1, 'm_P')
      | port_label('input', 2, 'm_P0')
      | port_label('output', 2, 'W_p/.,P0')
      | port_label('input', 3, 'Fm')
      | port_label('output', 3, 'm_x','interpreter','tex')
  W_body/.,P1 : Outport  VectorParamsAs1DForOutWhenUnconnected=off
  m_x : Outport  Port=2  VectorParamsAs1DForOutWhenUnconnected=off
  m_P2 : Outport  Port=3
  m_P3 : Outport  Port=4
  wires:
  Prismatic joint + configuration/1(m_P) -> Multi port rigid body/1(in1)
  Multi port rigid body/1(out1) -> Prismatic joint + configuration/1(W_./p,P)
  m_P1/1 -> Prismatic joint + configuration/2(m_P0)
  Fm/1 -> Prismatic joint + configuration/3(Fm)
  Prismatic joint + configuration/2(W_p/.,P0) -> W_body/.,P1/1
  Prismatic joint + configuration/3(m_x) -> m_x/1
  W_./body,P2/1 -> Multi port rigid body/2(in2)
  Multi port rigid body/2(out2) -> m_P2/1
  W_./body,P3/1 -> Multi port rigid body/3(in3)
  Multi port rigid body/3(out3) -> m_P3/1

== system SDTlibV1/Predefined subsystems/Multi port rigid body + revolute joint ==
  m_P1|p : Inport
  Cm : Inport  Port=2
  W_./body,P2|a : Inport  Port=3
  W_./body,P3|a : Inport  Port=4
  Multi port rigid body : Subsystem  mask(Multi-port rigid body (6nx6n)){m=m, Ig=Ignew, OG=OG, n=3, numinv=1, OP1=[0;0;0], OP2=[0;0;0.5], OP3=[0;0;0.25], OP4=[0;12;0], OP5=[0;0;0]}
      mask prompts: m "Mass (Kg)"; Ig "Inertia (at G, Kg m^2)"; OG "OG (3x1 vector, m)"; n "Number of ports"; numinv "Port to be inverted"; OP1 "OP1 (3x1 vector, m)"; OP2 "OP2 (3x1 vector, m)"; OP3 "OP3 (3x1 vector, m)"; OP4 "OP4 (3x1 vector, m)"; OP5 "OP5 (3x1 vector,m)"
      mask help:
      | 6nx6n dynamic model of a rigid body at n given points (ports) between wrenches applied at the n points (input) and acceleration twists at these points (output).
      |
      | 0: the reference point
      | G: the center of mass
      | Pi (i=1:n): the n given connection points (n<6).
      |
      | All parameters are expressed in the body frame.
      | Each parameter can be an uncertain parameter declared with "ureal"
      |
      | The 6x6 channel associated to one port can be inverted: then the input of this channel is the acceleration twist imposed at this point and the output is the wrench applied by this body.
      mask init:
      | MultiPortRigidBodyAug
      mask Help: web('Docmultiportrigidbody.html','-browser','-browser')
      mask TypeOptions n: 1 | 2 | 3 | 4 | 5
      mask TypeOptions numinv: 1 | 2 | 3 | 4 | 5
      mask DialogControl ParameterGroupVar Prompt: Main parameters
      mask DialogControl port1 Prompt: Port #1
      mask DialogControl port2 Prompt: #2
      mask DialogControl port3 Prompt: #3
      mask DialogControl port4 Prompt: #4
      mask DialogControl port5 Prompt: #5
      mask Display:
      | disp('Multi-port\n rigid body\n [18(n-1)+6]x[6(n-1)+18])')
      | if n==1,
      |     if numinv==1,
      |         port_label('input', 1,'m_P')
      |         port_label('output',1,'W_body/.,P')
      |     else
      |         port_label('input', 1,'W_./body,P')
      |         port_label('output',1,'m_P')
      |     end
      | else
      |     for ii=1:n
      |         if numinv==ii,
      |             port_label('output',ii,['W_body/.,P',num2str(ii)])
      |             port_label('input', ii,['m_P',num2str(ii)])
      |         else
      |             port_label('input', ii,['W_./body,P',num2str(ii)])
      |             port_label('output',ii,['m_P',num2str(ii)])
      |         end
      |     end
      | end
  Revolute joint + configuration : Subsystem  mask(Revolute joint){ra=ra_norm, Jr=Jr, theta=theta}
      mask prompts: ra "Direction of the joint in the local frame (3x1 vector)"; Jr "Rotor inertia (kg.m^2)"; theta "Angular configuration (rad)"
      mask help:
      | This block implement the TITOP model of of a revolute joint.
      | The last channel is the transfer between the torque applied inside the joint by the input shaft to the output shaft and the relative angular acceleration of the output shaft w.r.t the input shaft.
      |
      | Angular configuration can be a vayring parameter: Ex:
      | ureal('NAME',0,'Range',[-pi pi])
      |
      | Then, ULINEARIZE will provide a model involving the block named "tan_NAME_div4";
      mask init:
      | pass=ra2DCMi(ra);
      | ran=[ra(1);ra(2);ra(3)]/norm(ra);
      mask Help: web('DocRevoluteJoint_configuration.html','-browser','-browser')
      mask Display:
      | disp('Revolute joint\nTITOP model\n+ angle configuration')
      | port_label('input', 1, 'W_./r_out|a')
      | port_label('output', 1, 'm_out|a')
      | port_label('input', 2, 'm_in|p')
      | port_label('output', 2, 'W_r_in/.|p')
      | port_label('input', 3, 'Cm')
      | port_label('output', 3, 'm_\theta','interpreter','tex')
  W_body/.,P1|p : Outport  VectorParamsAs1DForOutWhenUnconnected=off
  m_theta : Outport  Port=2  VectorParamsAs1DForOutWhenUnconnected=off
  m_P2|a : Outport  Port=3
  m_P3|a : Outport  Port=4
  wires:
  Revolute joint + configuration/1(m_out|a) -> Multi port rigid body/1(in1)
  Multi port rigid body/1(out1) -> Revolute joint + configuration/1(W_./r_out|a)
  m_P1|p/1 -> Revolute joint + configuration/2(m_in|p)
  Cm/1 -> Revolute joint + configuration/3(Cm)
  Revolute joint + configuration/2(W_r_in/.|p) -> W_body/.,P1|p/1
  Revolute joint + configuration/3(m_theta) -> m_theta/1
  W_./body,P2|a/1 -> Multi port rigid body/2(in2)
  Multi port rigid body/2(out2) -> m_P2|a/1
  W_./body,P3|a/1 -> Multi port rigid body/3(in3)
  Multi port rigid body/3(out3) -> m_P3|a/1

== system SDTlibV1/Predefined subsystems/TITOP flexible beam +revolute joint ==
  W_./body,C|a : Inport  PortDimensions=6
  Cm : Inport  Port=2
  m_P|p : Inport  Port=3  PortDimensions=18
  Demux : Demux  Outputs=[18 6]
      settings: DisplayOption=none
  Mux : Mux  Inputs=[6 18]
  Revolute joint + configuration : Subsystem  mask(Revolute joint){ra=ra, Jr=Jr, theta=theta}
      mask prompts: ra "Direction of the joint in the local frame (3x1 vector)"; Jr "Rotor inertia (kg.m^2)"; theta "Angular configuration (rad)"
      mask help:
      | This block implement the TITOP model of of a revolute joint.
      | The last channel is the transfer between the torque applied inside the joint by the input shaft to the output shaft and the relative angular acceleration of the output shaft w.r.t the input shaft.
      |
      | Angular configuration can be a vayring parameter: Ex:
      | ureal('NAME',0,'Range',[-pi pi])
      |
      | Then, ULINEARIZE will provide a model involving the block named "tan_NAME_div4";
      mask init:
      | pass=ra2DCMi(ra);
      | ran=[ra(1);ra(2);ra(3)]/norm(ra);
      mask Help: web('DocRevoluteJoint_configuration.html','-browser','-browser')
      mask Display:
      | disp('Revolute joint\nTITOP model\n+ angle configuration')
      | port_label('input', 1, 'W_./r_out|a')
      | port_label('output', 1, 'm_out|a')
      | port_label('input', 2, 'm_in|p')
      | port_label('output', 2, 'W_r_in/.|p')
      | port_label('input', 3, 'Cm')
      | port_label('output', 3, 'm_\theta','interpreter','tex')
  Uncertain State Space : RCTblocks/Uncertain State Space  Tag=USS  USystem=TITOPBEAM  UValue=[]  X0=[]  uX0=[]
  m_C|a : Outport  VectorParamsAs1DForOutWhenUnconnected=off
  m_theta : Outport  Port=2  VectorParamsAs1DForOutWhenUnconnected=off
  W_body/.,P|p : Outport  Port=3  VectorParamsAs1DForOutWhenUnconnected=off
  wires:
  Cm/1 -> Revolute joint + configuration/3(Cm)
  Revolute joint + configuration/1(m_out|a) -> Mux/2
  Revolute joint + configuration/2(W_r_in/.|p) -> W_body/.,P|p/1
  Revolute joint + configuration/3(m_theta) -> m_theta/1
  m_P|p/1 -> Revolute joint + configuration/2(m_in|p)
  Demux/2 -> Revolute joint + configuration/1(W_./r_out|a)
  Demux/1 -> m_C|a/1
  W_./body,C|a/1 -> Mux/1
  Mux/1 -> Uncertain State Space/1
  Uncertain State Space/1 -> Demux/1

== system SDTlibV1/Space  subsystems/2 axis (x-y) Fast Steering Mirror (FSM) ==
  m_in : Inport  PortDimensions=18
  THETA_xy_cmd : Inport  Port=2  PortDimensions=2
  Demux : Demux  Outputs=2
  Demux1 : Demux  Outputs=3
  Demux2 : Demux  Outputs=3
  Gain : Gain  Gain=FSM.k
  Gain1 : Gain  Gain=FSM.d
  Gain2 : Gain  Gain=FSM.d
  Gain3 : Gain  Gain=FSM.k
  Ground : Ground
  Multi port rigid body + revolute joint1 : Subsystem  mask(Multi-port rigid body with revolute joint (18n-9)x(6n+15)){m=FSM.m, Ig=FSM.IatG, OG=[0;0;0], n=2, OP1=[0;0;0], OP2=[0;0;0], OP3=[0;0;0.25], OP4=[0;12;0], OP5=[0;0;0], ra=[1;0;0], theta=0}
      mask prompts: m "Mass (kg)"; Ig "Inertia at G in Ra (kg.m^2)"; OG "OG (3x1 vector in Ra)  (m)"; n "n (number of connection points)"; OP1 "OP1 (3x1 vector in Ra) (m)"; OP2 "OP2 (3x1 vector in Ra) (m)"; OP3 "OP3 (3x1 vector in Ra) (m)"; OP4 "OP4 (3x1 vector in Ra) (m)"; OP5 "OP5 (3x1 vector in Ra) (m)"; ra "ra (joint axis) (3x1 vector)"; theta "Angular configuration (rad)"
      mask help:
      | Computes the (18n-9)x(6n+13) model :
      | - 6x18 transfer from the motion vector to the wrench applied by this body to a parent body at port P1 through a revolute joint,
      | - the 3x1 channel :
      |               * from  the  joint torque applied by the input (parent) shaft to the output (body) shaft
      |               * to the relative motion vector of the output shaft w.r.t the input shaft ([thetaddot;thetadot;theta]),
      | - (n-1) 18x6 transfers from the wrenches applied to this body to the motion vectors at ports P2,P3,..,
      |
      | Input/Output of port P1 are expressed in the parent frame Rp
      | Input/Output of ports P2,P3,... are expressed in the body frame Ra.
      |
      | O: the body reference point
      | G: the center of mass
      | Pi (i=1:n): the n given connection points or ports (n<6).
      | ra: direction of the revolute joint in the Rp (or Ra)
      | theta: angular configuration of the joint (Ra is obtained from Rp by a rotation of theta around ra).
      |
      | All parameters must be expressed in the body frame Ra.
      | Each parameter can be an uncertain parameter declared with the function ureal (except ra)
      |
      | Rk: if "theta" field is: ureal('NAME',0,'Range',[-pi pi])
      | then, ULINEARIZE will provide a model involving the block named "tan_NAME_div4";
      mask init:
      | MultiPortRigidBodyRevAug
      mask Help: web('DocMultiportRigidBodyRevolute.html','-browser','-browser')
      mask TypeOptions n: 1 | 2 | 3 | 4 | 5
      mask DialogControl ParameterGroupVar Prompt: Rigid body parameter
      mask DialogControl port1 Prompt: #1
      mask DialogControl port2 Prompt: #2
      mask DialogControl port3 Prompt: #3
      mask DialogControl port4 Prompt: #4
      mask DialogControl port5 Prompt: #5
      mask DialogControl JointParameters Prompt: Revolute joint parameters
      mask Display:
      | disp('Multi-port\n rigid body\n+ revolute joint \n(18n-9)x(6n+13)')
      | 
      | port_label('input', 1,'m_P1|p')
      | port_label('output',1,'W_body/.,P1|p')
      | port_label('input', 2,'Cm_at_P1')
      | port_label('output',2,'m_\theta at P1','interpreter','tex')
      | 
      | if n>1
      |     for i=2:n
      |         port_label('input', i+1,['W_./body,P',num2str(i),'|a'])
      |         port_label('output',i+1,['m_P',num2str(i),'|a'])
      |     end
      | end
  Mux : Mux  Inputs=2
  Mux1 : Mux  Inputs=2
  Mux2 : Mux  Inputs=2
  Revolute joint + configuration : Subsystem  mask(Revolute joint){ra=[0;1;0], Jr=1e-9, theta=0}
      mask prompts: ra "Direction of the joint in the local frame (3x1 vector)"; Jr "Rotor inertia (kg.m^2)"; theta "Angular configuration (rad)"
      mask help:
      | This block implement the TITOP model of of a revolute joint.
      | The last channel is the transfer between the torque applied inside the joint by the input shaft to the output shaft and the relative angular acceleration of the output shaft w.r.t the input shaft.
      |
      | Angular configuration can be a vayring parameter: Ex:
      | ureal('NAME',0,'Range',[-pi pi])
      |
      | Then, ULINEARIZE will provide a model involving the block named "tan_NAME_div4";
      mask init:
      | pass=ra2DCMi(ra);
      | ran=[ra(1);ra(2);ra(3)]/norm(ra);
      mask Help: web('DocRevoluteJoint_configuration.html','-browser','-browser')
      mask Display:
      | disp('Revolute joint\nTITOP model\n+ angle configuration')
      | port_label('input', 1, 'W_./r_out|a')
      | port_label('output', 1, 'm_out|a')
      | port_label('input', 2, 'm_in|p')
      | port_label('output', 2, 'W_r_in/.|p')
      | port_label('input', 3, 'Cm')
      | port_label('output', 3, 'm_\theta','interpreter','tex')
  Sum : Sum  Inputs=|+-
  Sum1 : Sum  Inputs=-+|
  Sum2 : Sum  Inputs=+-
  Sum3 : Sum  Inputs=+-
  W_FSM/.,P : Outport
  THETAddot_xy : Outport  Port=2
  THETAdot_xy : Outport  Port=3
  THETA_xy : Outport  Port=4
  Xddot_FSM : Outport  Port=5
  wires:
  Gain2/1 -> Sum/2
  Gain3/1 -> Sum/1
  Demux/1 -> Sum3/1
  Sum3/1 -> Gain3/1
  Demux/2 -> Sum2/1
  Sum2/1 -> Gain/1
  Gain/1 -> Sum1/2
  Gain1/1 -> Sum1/1
  Sum1/1 -> Revolute joint + configuration/3(Cm)
  Demux2/3 -> Mux2/1, Sum3/2
  Sum/1 -> Multi port rigid body + revolute joint1/2(Cm)
  Demux1/3 -> Mux2/2, Sum2/2
  Mux2/1 -> THETA_xy/1
  Mux1/1 -> THETAdot_xy/1
  Demux1/2 -> Mux1/2, Gain1/1
  Demux2/2 -> Mux1/1, Gain2/1
  Ground/1 -> Multi port rigid body + revolute joint1/3(W_./body,P2|a)
  Multi port rigid body + revolute joint1/1(W_body/.,P1|p) -> Revolute joint + configuration/1(W_./r_out|a)
  Revolute joint + configuration/1(m_out|a) -> Multi port rigid body + revolute joint1/1(m_P1|p)
  Multi port rigid body + revolute joint1/3(m_P2|a) -> Xddot_FSM/1
  Mux/1 -> THETAddot_xy/1
  Revolute joint + configuration/3(m_theta) -> Demux1/1
  Revolute joint + configuration/2(W_r_in/.|p) -> W_FSM/.,P/1
  m_in/1 -> Revolute joint + configuration/2(m_in|p)
  Multi port rigid body + revolute joint1/2(m_theta) -> Demux2/1
  THETA_xy_cmd/1 -> Demux/1
  Demux1/1 -> Mux/2
  Demux2/1 -> Mux/1
